simulink library "MK_H"  (R2025a)
settings: Solver=VariableStepAuto  StartTime=0.0  StopTime=10.0  RelTol=1e-3
settings Model: Creator=Szalay  LastModifiedBy=Szalay

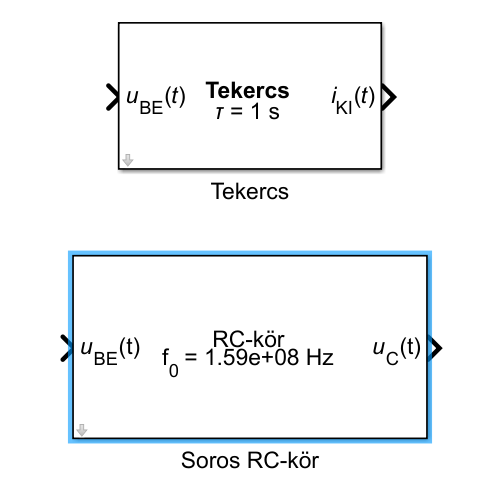
[thumbnail: Simulink's stored preview of the top-level diagram]
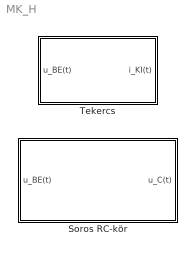
== system MK_H ==
  Soros RC-kör : Subsystem  mask(Soros RC-kör){R=1, C=1e-9, u_C0=0}
      mask prompts: R "Ellenállás (Ohm)"; C "Kapacitás (F)"; u_C0 "A kapacitáson eső feszültség kezdeti értéke (V)"
      mask help: Sorba kapcsolt ellenállás és kapaqcitás modellje.
      mask DialogControl ParameterGroupVar Prompt: Modellparaméterek
      mask DialogControl Container3 Prompt: Kezdeti érték
      mask Display:
      | % Csatlakozók
      | port_label('input', 1, '{\itu}_{BE}(t)', 'texmode', 'on');
      | port_label('output', 1, '{\itu}_C(t)', 'texmode', 'on');
      | 
      | R = str2double(get_param(gcb, 'R'));
      | C = str2double(get_param(gcb, 'C'));
      | 
      | % Felirat
      | text(0.5, 0.5, ...
      |     sprintf('RC-kör\nf_0 = %.3g Hz', 1/(R*C)/(2*pi)), ...
      |     'HorizontalAlignment', 'center', ...
      |     'Interpreter', 'tex' ...
      |     );
  Tekercs : Subsystem  mask(Tekercsmodell){R=2, L=2e-3, i_0=0.5}
      mask prompts: R "Ellenállás (Ohm)"; L "Öninduktivitás (H)"; i_0 "Az áramerősség kezdeti értéke (A)"
      mask help: Lineáris mágnesezettségű tekercs (RL-tag) modellje.
      mask DialogControl ParameterGroupVar Prompt: Modellparaméterek
      mask DialogControl Container3 Prompt: Kezdeti érték
      mask Display:
      | %L = get_param(gcb, 'L');
      | %R = get_param(gcb, 'R');
      | 
      | % Az időállandó
      | tau = 1;
      | 
      | text( ...
      |     0.5, 0.5, sprintf('{\\bfTekercs}\n{\\it\\tau} = %g s', tau), ...
      |     'HorizontalAlignment', 'center', ...
      |     'Interpreter', 'tex' ...
      |     );
      | 
      | port_label('input', 1, '{\itu}_{BE}({\itt})', 'texmode', 'on');
      | port_label('output', 1, '{\iti}_{KI}({\itt})', 'texmode', 'on');

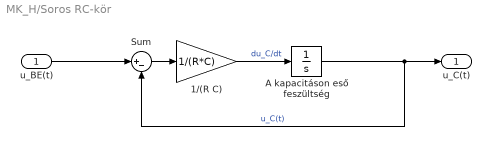
== system MK_H/Soros RC-kör ==
  u_BE(t) : Inport
  1/(R C) : Gain  Gain=1/(R*C)
  A kapacitáson eső feszültség : Integrator
  Sum : Sum  Inputs=|+-
  u_C(t) : Outport
  wires:
  A kapacitáson eső feszültség/1 -> u_C(t)/1, Sum/2  "u_C(t)"
  Sum/1 -> 1/(R C)/1
  u_BE(t)/1 -> Sum/1
  1/(R C)/1 -> A kapacitáson eső feszültség/1  "du_C/dt"

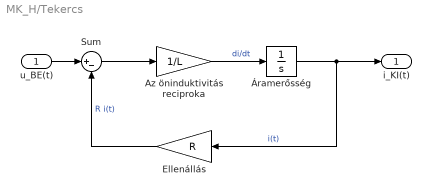
== system MK_H/Tekercs ==
  u_BE(t) : Inport
  Az öninduktivitás reciproka : Gain  Gain=1/L
  Ellenállás : Gain  Gain=R
  Sum : Sum  Inputs=|+-
  Áramerősség : Integrator  InitialCondition=i_0
  i_KI(t) : Outport
  wires:
  Az öninduktivitás reciproka/1 -> Áramerősség/1  "di/dt"
  u_BE(t)/1 -> Sum/1
  Áramerősség/1 -> i_KI(t)/1, Ellenállás/1  "i(t)"
  Ellenállás/1 -> Sum/2  "R i(t)"
  Sum/1 -> Az öninduktivitás reciproka/1
